simulink model "v12_SR_flipflops"  (R2019b)
settings: Solver=FixedStepAuto  StartTime=0.0  StopTime=inf  FixedStep=1  MaxStep=1  RelTol=1e-3
settings Model: Creator=MARAT  LastModifiedBy=Marat
settings SFSimCC: CustomCodeUndefinedFunction=UseInterfaceOnly

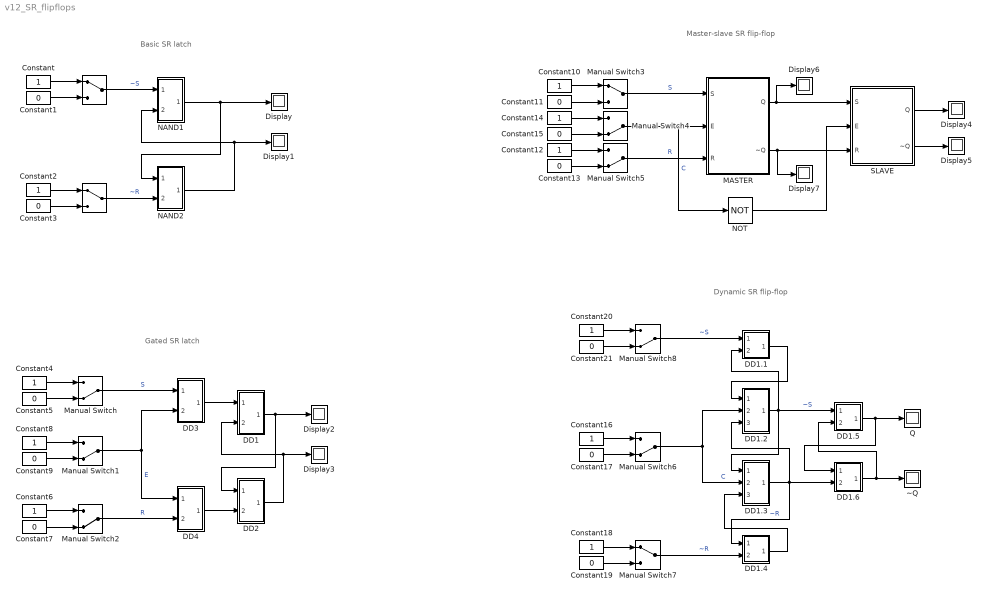
== system v12_SR_flipflops ==
  note: Dynamic SR flip-flop
  note: Master-slave SR flip-flop
  note: Basic SR latch
  note: Gated SR latch
  " " : ManualSwitch
  " " : ManualSwitch
  Constant{,2,4,6,8,10,12,14,16,18,20} (11 alike) : Constant  OutDataTypeStr=boolean
  Constant{1,3,5,7,9,11,13,15,17,19,21} (11 alike) : Constant  Value=0  OutDataTypeStr=boolean
  DD1 : Subsystem
      mask Display: disp('&~');
  DD1.1 : Subsystem
      mask Display: disp('&~');
  DD1.2 : Subsystem
      mask Display: disp('&~');
  DD1.3 : Subsystem
      mask Display: disp('&~');
  DD1.4 : Subsystem
      mask Display: disp('&~');
  DD1.5 : Subsystem
      mask Display: disp('&~');
  DD1.6 : Subsystem
      mask Display: disp('&~');
  DD2 : Subsystem
      mask Display: disp('&~');
  DD3 : Subsystem
      mask Display: disp('&~');
  DD4 : Subsystem
      mask Display: disp('&~');
  Display{,1..7} (8 alike) : Display
  MASTER : Subsystem
      mask Display: disp('SR \nlatch \ngated');
  Manual Switch{,1..2,4..6,8} (7 alike) : ManualSwitch  CurrentSetting=0
  Manual Switch3 : ManualSwitch
  Manual Switch7 : ManualSwitch
  NAND1 : Subsystem
      mask Display: disp('&~');
  NAND2 : Subsystem
      mask Display: disp('&~');
  NOT : Logic  Operator=NOT  IconShape=distinctive  AllPortsSameDT=off  OutDataTypeStr=boolean
  Q : Display
  SLAVE : Subsystem
      mask Display: disp('SR \nlatch \ngated');
  ~Q : Display
  wires:
  DD1.5/1(Out1) -> DD1.6/1(In1), Q/1
  DD1.3/1(Out1) -> DD1.4/1(In1), DD1.6/2(In2), DD1.2/3(In3)  "~R"
  Constant18/1 -> Manual Switch7/1
  Constant19/1 -> Manual Switch7/2
  Manual Switch7/1 -> DD1.4/2(In2)  "~R"
  Constant16/1 -> Manual Switch6/1
  Constant17/1 -> Manual Switch6/2
  DD1.6/1(Out1) -> DD1.5/2(In2), ~Q/1
  Manual Switch6/1 -> DD1.2/2(In2), DD1.3/2(In2)  "C"
  Constant21/1 -> Manual Switch8/2
  Constant20/1 -> Manual Switch8/1
  Manual Switch8/1 -> DD1.1/1(In1)  "~S"
  DD1.2/1(Out1) -> DD1.1/2(In2), DD1.5/1(In1), DD1.3/1(In1)  "~S"
  DD1.1/1(Out1) -> DD1.2/1(In1)
  DD1.4/1(Out1) -> DD1.3/3(In3)
  Constant10/1 -> Manual Switch3/1
  MASTER/2(~Q) -> Display7/1, SLAVE/3(R)
  MASTER/1(Q) -> SLAVE/1(S), Display6/1
  Manual Switch3/1 -> MASTER/1(S)  "S"
  SLAVE/2(~Q) -> Display5/1
  Constant13/1 -> Manual Switch5/2
  Constant15/1 -> Manual Switch4/2
  Manual Switch4/1 -> NOT/1, MASTER/2(E)  "C"
  Manual Switch5/1 -> MASTER/3(R)  "R"
  Constant12/1 -> Manual Switch5/1
  NOT/1 -> SLAVE/2(E)
  Constant11/1 -> Manual Switch3/2
  SLAVE/1(Q) -> Display4/1
  Constant14/1 -> Manual Switch4/1
  NAND1/1(Out1) -> NAND2/1(In1), Display/1
  Constant9/1 -> Manual Switch1/2
  Constant2/1 -> " "/1
  Manual Switch2/1 -> DD4/2(In2)  "R"
  " "/1 -> NAND2/2(In2)  "~R"
  DD3/1(Out1) -> DD1/1(In1)
  Constant5/1 -> Manual Switch/2
  Constant8/1 -> Manual Switch1/1
  Manual Switch1/1 -> DD4/1(In1), DD3/2(In2)  "E"
  Constant1/1 -> " "/2
  NAND2/1(Out1) -> NAND1/2(In2), Display1/1
  DD2/1(Out1) -> Display3/1, DD1/2(In2)
  DD4/1(Out1) -> DD2/2(In2)
  DD1/1(Out1) -> Display2/1, DD2/1(In1)
  Constant6/1 -> Manual Switch2/1
  Constant3/1 -> " "/2
  Constant7/1 -> Manual Switch2/2
  Manual Switch/1 -> DD3/1(In1)  "S"
  Constant4/1 -> Manual Switch/1
  Constant/1 -> " "/1
  " "/1 -> NAND1/1(In1)  "~S"

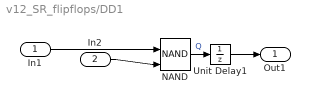
== system v12_SR_flipflops/DD1 ==
  In1 : Inport
  In2 : Inport  Port=2
  NAND : Logic  Operator=NAND  IconShape=distinctive  AllPortsSameDT=off  OutDataTypeStr=boolean
  Unit Delay1 : UnitDelay  SampleTime=-1  HasFrameUpgradeWarning=on
  Out1 : Outport
  wires:
  NAND/1 -> Unit Delay1/1  "Q"
  Unit Delay1/1 -> Out1/1
  In1/1 -> NAND/1
  In2/1 -> NAND/2

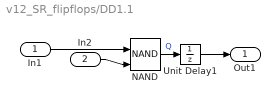
== system v12_SR_flipflops/DD1.1 ==
  In1 : Inport
  In2 : Inport  Port=2
  NAND : Logic  Operator=NAND  IconShape=distinctive  AllPortsSameDT=off  OutDataTypeStr=boolean
  Unit Delay1 : UnitDelay  SampleTime=-1  HasFrameUpgradeWarning=on
  Out1 : Outport
  wires:
  NAND/1 -> Unit Delay1/1  "Q"
  Unit Delay1/1 -> Out1/1
  In1/1 -> NAND/1
  In2/1 -> NAND/2

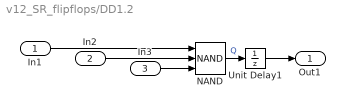
== system v12_SR_flipflops/DD1.2 ==
  In1 : Inport
  In2 : Inport  Port=2
  In3 : Inport  Port=3
  NAND : Logic  Operator=NAND  Inputs=3  IconShape=distinctive  AllPortsSameDT=off  OutDataTypeStr=boolean
  Unit Delay1 : UnitDelay  SampleTime=-1  HasFrameUpgradeWarning=on
  Out1 : Outport
  wires:
  In3/1 -> NAND/3
  In2/1 -> NAND/2
  In1/1 -> NAND/1
  Unit Delay1/1 -> Out1/1
  NAND/1 -> Unit Delay1/1  "Q"

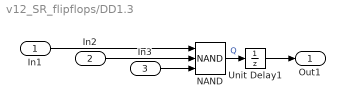
== system v12_SR_flipflops/DD1.3 ==
  In1 : Inport
  In2 : Inport  Port=2
  In3 : Inport  Port=3
  NAND : Logic  Operator=NAND  Inputs=3  IconShape=distinctive  AllPortsSameDT=off  OutDataTypeStr=boolean
  Unit Delay1 : UnitDelay  SampleTime=-1  HasFrameUpgradeWarning=on
  Out1 : Outport
  wires:
  NAND/1 -> Unit Delay1/1  "Q"
  Unit Delay1/1 -> Out1/1
  In1/1 -> NAND/1
  In2/1 -> NAND/2
  In3/1 -> NAND/3

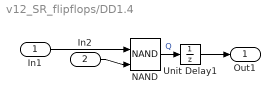
== system v12_SR_flipflops/DD1.4 ==
  In1 : Inport
  In2 : Inport  Port=2
  NAND : Logic  Operator=NAND  IconShape=distinctive  AllPortsSameDT=off  OutDataTypeStr=boolean
  Unit Delay1 : UnitDelay  SampleTime=-1  HasFrameUpgradeWarning=on
  Out1 : Outport
  wires:
  NAND/1 -> Unit Delay1/1  "Q"
  Unit Delay1/1 -> Out1/1
  In1/1 -> NAND/1
  In2/1 -> NAND/2

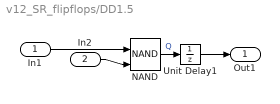
== system v12_SR_flipflops/DD1.5 ==
  In1 : Inport
  In2 : Inport  Port=2
  NAND : Logic  Operator=NAND  IconShape=distinctive  AllPortsSameDT=off  OutDataTypeStr=boolean
  Unit Delay1 : UnitDelay  SampleTime=-1  HasFrameUpgradeWarning=on
  Out1 : Outport
  wires:
  In2/1 -> NAND/2
  In1/1 -> NAND/1
  Unit Delay1/1 -> Out1/1
  NAND/1 -> Unit Delay1/1  "Q"

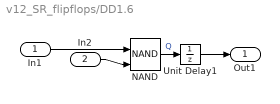
== system v12_SR_flipflops/DD1.6 ==
  In1 : Inport
  In2 : Inport  Port=2
  NAND : Logic  Operator=NAND  IconShape=distinctive  AllPortsSameDT=off  OutDataTypeStr=boolean
  Unit Delay1 : UnitDelay  SampleTime=-1  HasFrameUpgradeWarning=on
  Out1 : Outport
  wires:
  NAND/1 -> Unit Delay1/1  "Q"
  Unit Delay1/1 -> Out1/1
  In1/1 -> NAND/1
  In2/1 -> NAND/2

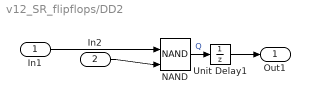
== system v12_SR_flipflops/DD2 ==
  In1 : Inport
  In2 : Inport  Port=2
  NAND : Logic  Operator=NAND  IconShape=distinctive  AllPortsSameDT=off  OutDataTypeStr=boolean
  Unit Delay1 : UnitDelay  SampleTime=-1  HasFrameUpgradeWarning=on
  Out1 : Outport
  wires:
  In2/1 -> NAND/2
  In1/1 -> NAND/1
  Unit Delay1/1 -> Out1/1
  NAND/1 -> Unit Delay1/1  "Q"

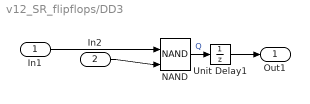
== system v12_SR_flipflops/DD3 ==
  In1 : Inport
  In2 : Inport  Port=2
  NAND : Logic  Operator=NAND  IconShape=distinctive  AllPortsSameDT=off  OutDataTypeStr=boolean
  Unit Delay1 : UnitDelay  SampleTime=-1  HasFrameUpgradeWarning=on
  Out1 : Outport
  wires:
  In2/1 -> NAND/2
  In1/1 -> NAND/1
  Unit Delay1/1 -> Out1/1
  NAND/1 -> Unit Delay1/1  "Q"

== system v12_SR_flipflops/DD4 ==
  In1 : Inport
  In2 : Inport  Port=2
  NAND : Logic  Operator=NAND  IconShape=distinctive  AllPortsSameDT=off  OutDataTypeStr=boolean
  Unit Delay1 : UnitDelay  SampleTime=-1  HasFrameUpgradeWarning=on
  Out1 : Outport
  wires:
  NAND/1 -> Unit Delay1/1  "Q"
  Unit Delay1/1 -> Out1/1
  In1/1 -> NAND/1
  In2/1 -> NAND/2

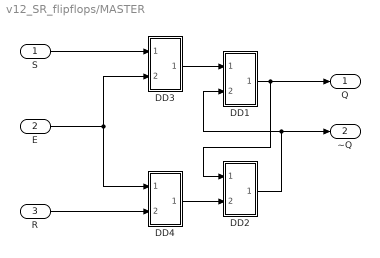
== system v12_SR_flipflops/MASTER ==
  S : Inport
  E : Inport  Port=2
  R : Inport  Port=3
  DD1 : Subsystem
      mask Display: disp('&~');
  DD2 : Subsystem
      mask Display: disp('&~');
  DD3 : Subsystem
      mask Display: disp('&~');
  DD4 : Subsystem
      mask Display: disp('&~');
  Q : Outport
  ~Q : Outport  Port=2
  wires:
  DD3/1(Out1) -> DD1/1(In1)
  DD1/1(Out1) -> Q/1, DD2/1(In1)
  E/1 -> DD4/1(In1), DD3/2(In2)
  S/1 -> DD3/1(In1)
  DD4/1(Out1) -> DD2/2(In2)
  R/1 -> DD4/2(In2)
  DD2/1(Out1) -> ~Q/1, DD1/2(In2)

== system v12_SR_flipflops/NAND1 ==
  In1 : Inport
  In2 : Inport  Port=2
  NAND : Logic  Operator=NAND  IconShape=distinctive  AllPortsSameDT=off  OutDataTypeStr=boolean
  Unit Delay1 : UnitDelay  SampleTime=-1  HasFrameUpgradeWarning=on
  Out1 : Outport
  wires:
  NAND/1 -> Unit Delay1/1  "Q"
  Unit Delay1/1 -> Out1/1
  In1/1 -> NAND/1
  In2/1 -> NAND/2

== system v12_SR_flipflops/NAND2 ==
  In1 : Inport
  In2 : Inport  Port=2
  NAND : Logic  Operator=NAND  IconShape=distinctive  AllPortsSameDT=off  OutDataTypeStr=boolean
  Unit Delay1 : UnitDelay  SampleTime=-1  HasFrameUpgradeWarning=on
  Out1 : Outport
  wires:
  In2/1 -> NAND/2
  In1/1 -> NAND/1
  Unit Delay1/1 -> Out1/1
  NAND/1 -> Unit Delay1/1  "Q"

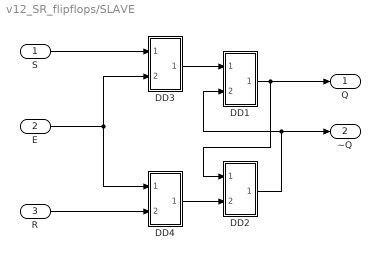
== system v12_SR_flipflops/SLAVE ==
  S : Inport
  E : Inport  Port=2
  R : Inport  Port=3
  DD1 : Subsystem
      mask Display: disp('&~');
  DD2 : Subsystem
      mask Display: disp('&~');
  DD3 : Subsystem
      mask Display: disp('&~');
  DD4 : Subsystem
      mask Display: disp('&~');
  Q : Outport
  ~Q : Outport  Port=2
  wires:
  DD2/1(Out1) -> DD1/2(In2), ~Q/1
  R/1 -> DD4/2(In2)
  DD4/1(Out1) -> DD2/2(In2)
  S/1 -> DD3/1(In1)
  E/1 -> DD3/2(In2), DD4/1(In1)
  DD1/1(Out1) -> DD2/1(In1), Q/1
  DD3/1(Out1) -> DD1/1(In1)

== system v12_SR_flipflops/MASTER/DD1 ==
  In1 : Inport
  In2 : Inport  Port=2
  NAND : Logic  Operator=NAND  IconShape=distinctive  AllPortsSameDT=off  OutDataTypeStr=boolean
  Unit Delay1 : UnitDelay  SampleTime=-1  HasFrameUpgradeWarning=on
  Out1 : Outport
  wires:
  NAND/1 -> Unit Delay1/1  "Q"
  Unit Delay1/1 -> Out1/1
  In1/1 -> NAND/1
  In2/1 -> NAND/2

== system v12_SR_flipflops/MASTER/DD2 ==
  In1 : Inport
  In2 : Inport  Port=2
  NAND : Logic  Operator=NAND  IconShape=distinctive  AllPortsSameDT=off  OutDataTypeStr=boolean
  Unit Delay1 : UnitDelay  SampleTime=-1  HasFrameUpgradeWarning=on
  Out1 : Outport
  wires:
  In2/1 -> NAND/2
  In1/1 -> NAND/1
  Unit Delay1/1 -> Out1/1
  NAND/1 -> Unit Delay1/1  "Q"

== system v12_SR_flipflops/MASTER/DD3 ==
  In1 : Inport
  In2 : Inport  Port=2
  NAND : Logic  Operator=NAND  IconShape=distinctive  AllPortsSameDT=off  OutDataTypeStr=boolean
  Unit Delay1 : UnitDelay  SampleTime=-1  HasFrameUpgradeWarning=on
  Out1 : Outport
  wires:
  In2/1 -> NAND/2
  In1/1 -> NAND/1
  Unit Delay1/1 -> Out1/1
  NAND/1 -> Unit Delay1/1  "Q"

== system v12_SR_flipflops/MASTER/DD4 ==
  In1 : Inport
  In2 : Inport  Port=2
  NAND : Logic  Operator=NAND  IconShape=distinctive  AllPortsSameDT=off  OutDataTypeStr=boolean
  Unit Delay1 : UnitDelay  SampleTime=-1  HasFrameUpgradeWarning=on
  Out1 : Outport
  wires:
  NAND/1 -> Unit Delay1/1  "Q"
  Unit Delay1/1 -> Out1/1
  In1/1 -> NAND/1
  In2/1 -> NAND/2

== system v12_SR_flipflops/SLAVE/DD1 ==
  In1 : Inport
  In2 : Inport  Port=2
  NAND : Logic  Operator=NAND  IconShape=distinctive  AllPortsSameDT=off  OutDataTypeStr=boolean
  Unit Delay1 : UnitDelay  SampleTime=-1  HasFrameUpgradeWarning=on
  Out1 : Outport
  wires:
  In2/1 -> NAND/2
  In1/1 -> NAND/1
  Unit Delay1/1 -> Out1/1
  NAND/1 -> Unit Delay1/1  "Q"

== system v12_SR_flipflops/SLAVE/DD2 ==
  In1 : Inport
  In2 : Inport  Port=2
  NAND : Logic  Operator=NAND  IconShape=distinctive  AllPortsSameDT=off  OutDataTypeStr=boolean
  Unit Delay1 : UnitDelay  SampleTime=-1  HasFrameUpgradeWarning=on
  Out1 : Outport
  wires:
  NAND/1 -> Unit Delay1/1  "Q"
  Unit Delay1/1 -> Out1/1
  In1/1 -> NAND/1
  In2/1 -> NAND/2

== system v12_SR_flipflops/SLAVE/DD3 ==
  In1 : Inport
  In2 : Inport  Port=2
  NAND : Logic  Operator=NAND  IconShape=distinctive  AllPortsSameDT=off  OutDataTypeStr=boolean
  Unit Delay1 : UnitDelay  SampleTime=-1  HasFrameUpgradeWarning=on
  Out1 : Outport
  wires:
  NAND/1 -> Unit Delay1/1  "Q"
  Unit Delay1/1 -> Out1/1
  In1/1 -> NAND/1
  In2/1 -> NAND/2

== system v12_SR_flipflops/SLAVE/DD4 ==
  In1 : Inport
  In2 : Inport  Port=2
  NAND : Logic  Operator=NAND  IconShape=distinctive  AllPortsSameDT=off  OutDataTypeStr=boolean
  Unit Delay1 : UnitDelay  SampleTime=-1  HasFrameUpgradeWarning=on
  Out1 : Outport
  wires:
  In2/1 -> NAND/2
  In1/1 -> NAND/1
  Unit Delay1/1 -> Out1/1
  NAND/1 -> Unit Delay1/1  "Q"
